simulink library "ReynoldsTHB"  (R2018b)
settings: Solver=ode45  StartTime=0.0  StopTime=10.0  RelTol=1e-3  EnableMultiTasking=on
libraries: carnot x2
settings Model: Creator=lena.frank  LastModifiedBy=drhf
settings DataIOCC: LimitDataPoints=on  SaveFormat=Array  SignalLoggingSaveFormat=ModelDataLogs
settings OptimizationCC: ExpressionDepthLimit=2147483647  LifeSpan=inf
settings DebuggingCC: UnderspecifiedInitializationDetection=Classic  MergeDetectMultiDrivingBlocksExec=none  SolverPrmCheckMsg=warning  FcnCallInpInsideContextMsg=warning  StateNameClashWarn=warning  SFUnexpectedBacktrackingDiag=warning  SFNoUnconditionalDefaultTransitionDiag=warning  SFExecutionAtInitializationDiag=none
settings HardwareCC: ProdBitPerPointer=32  ProdBitPerSizeT=32  ProdBitPerPtrDiffT=32  ProdLargestAtomicFloat=None  ProdIntDivRoundTo=Undefined  ProdEndianess=Unspecified  ProdWordSize=32  ProdHWDeviceType=32-bit Generic
settings ModelReferenceCC: PropagateSignalLabelsOutOfModel=off
settings SFSimCC: SimUseLocalCustomCode=off
settings RTWCC: RTWUseLocalCustomCode=off
settings CodeAppCC: StateflowObjectComments=on
settings GRTTargetCC: TargetLangStandard=C89/C90 (ANSI)  GeneratePreprocessorConditionals=Disable all  CombineOutputUpdateFcns=off  GRTInterface=on
settings ConfigComp: CovMetricSettings=dw  CovHtmlReporting=on  CovSaveCumulativeToWorkspaceVar=on  CovSaveSingleToWorkspaceVar=on  CovExternalEMLEnable=off

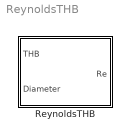
== system ReynoldsTHB ==
  ReynoldsTHB : Subsystem  mask(Reynolds THB){}
      mask help: Calculates the Reynolds number for pipes with round cross-section.
      mask Help: web(fullfile(path_carnot('help'),'ReynoldsTHB.html'),'-helpbrowser')

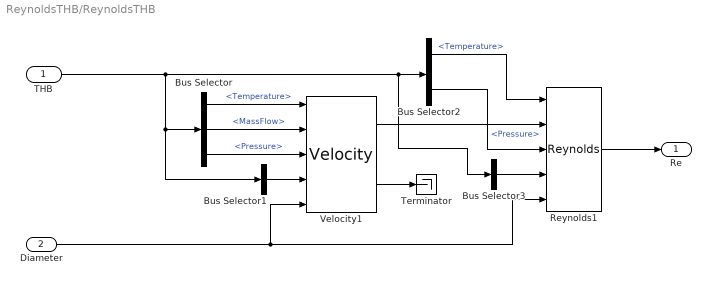
== system ReynoldsTHB/ReynoldsTHB ==
  THB : Inport
  Diameter : Inport  Port=2
  Bus Selector : BusSelector  OutputSignals=Temperature,MassFlow,Pressure
  Bus Selector1 : BusSelector  OutputSignals=FluidType,FluidMix  OutputAsBus=on
  Bus Selector2 : BusSelector  OutputSignals=Temperature,Pressure
  Bus Selector3 : BusSelector  OutputSignals=FluidType,FluidMix  OutputAsBus=on
  Reynolds1 : carnot/Basic/Hydraulics/Reynolds
      settings: SourceProductName=Carnot
  Terminator : Terminator
  Velocity1 : carnot/Basic/Hydraulics/Velocity
      settings: SourceProductName=Carnot
  Re : Outport
  wires:
  Diameter/1 -> Reynolds1/5, Velocity1/5
  Reynolds1/1 -> Re/1
  THB/1 -> Bus Selector3/1, Bus Selector2/1, Bus Selector1/1, Bus Selector/1
  Velocity1/2 -> Terminator/1
  Bus Selector2/2 -> Reynolds1/3  "<Pressure>"
  Bus Selector3/1 -> Reynolds1/4
  Bus Selector2/1 -> Reynolds1/1  "<Temperature>"
  Bus Selector1/1 -> Velocity1/4
  Bus Selector/3 -> Velocity1/3  "<Pressure>"
  Bus Selector/1 -> Velocity1/1  "<Temperature>"
  Bus Selector/2 -> Velocity1/2  "<MassFlow>"
  Velocity1/1 -> Reynolds1/2
